simulink model "kinematics_model_Vw_working"  (R2020b)
settings: Solver=VariableStepAuto  StartTime=0.0  StopTime=100  RelTol=1e-3
values from neighbouring files (symbols this model uses):
  theta0 = 5*pi/180    (= 0.0872664625997)    [Kinematics_model.m]    (also in Path_Planning.m)
  x0 = 0    [Kinematics_model.m]    (also in Path_Planning.m)
  xd = x(length(x))    [APF.m]    (also in Kinematics_model.m = 20; Path_Planning.m = 6)
  y0 = 0    [Kinematics_model.m]    (also in Path_Planning.m)
  yd = y(length(y))    [APF.m]    (also in Kinematics_model.m = 15; Path_Planning.m = 7)
libraries: simulink_extras x1, mobileRoboticsLib x1
settings Model: Creator=Roooooomaaaaaaaaaaaa  LastModifiedBy=Roooooomaaaaaaaaaaaa

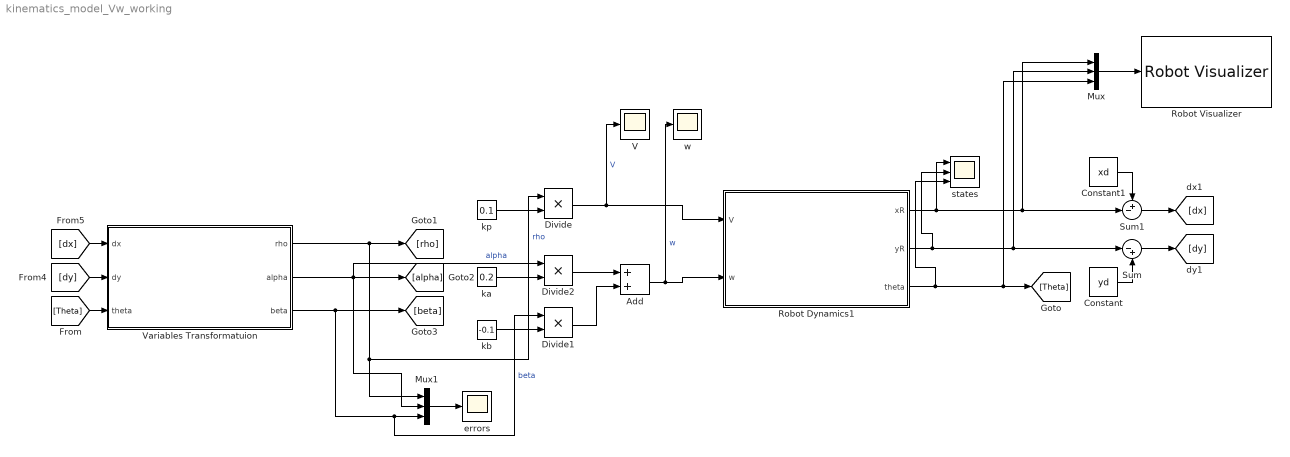
== system kinematics_model_Vw_working ==
  " Variables Transformatuion" : Subsystem
  Add : Sum
  Constant : Constant  Value=yd
  Constant1 : Constant  Value=xd
  Divide : Product  Inputs=**
  Divide1 : Product  Inputs=**
  Divide2 : Product  Inputs=**
  Mux : Mux  Inputs=3
  Mux1 : Mux  Inputs=3
  Robot Dynamics1 : Subsystem
  Robot Visualizer : mobileRoboticsLib/Environments/Robot Visualizer  robotRadius=r_w  showTrajectory=on  hasWaypoints=off  hasLidar=off  sensorOffset=[ 0, 0 ]  scanAngles=[ -pi/4, 0, pi/4 ]  hasObjDetector=off  objDetectorOffset=[ 0, 0 ]  objDetectorAngle=0  objDetectorFOV=pi/4  objDetectorMaxRange=5  objectColors=[ 1, 0, 0; 0, 1, 0; 0, 0, 1 ]  objectMarkers=s
  Sum : Sum  Inputs=|-+
  Sum1 : Sum  Inputs=+-|
  V : Scope
  errors : Scope
  ka : Constant  Value=0.2
  kb : Constant  Value=-0.1
  kp : Constant  Value=0.1
  states : Scope  NumInputPorts=3
  w : Scope
  wires:
  Mux/1 -> Robot Visualizer/1
  Divide1/1 -> Add/2
  Robot Dynamics1/2(yR) -> states/2, Sum/1, Mux/2
  Robot Dynamics1/3(theta) -> Mux/3, [Theta], states/3
  Divide2/1 -> Add/1
  [dy] -> " Variables Transformatuion"/2(dy)
  " Variables Transformatuion"/3(beta) -> [beta], Divide1/1, Mux1/3  "beta"
  " Variables Transformatuion"/2(alpha) -> Mux1/2, Divide2/1, [alpha]  "alpha"
  " Variables Transformatuion"/1(rho) -> Divide/1, Mux1/1, [rho]  "rho"
  kp/1 -> Divide/2
  ka/1 -> Divide2/2
  [Theta] -> " Variables Transformatuion"/3(theta)
  Sum1/1 -> [dx]
  Divide/1 -> V/1, Robot Dynamics1/1(V)  "V"
  Constant/1 -> Sum/2
  kb/1 -> Divide1/2
  Constant1/1 -> Sum1/1
  Sum/1 -> [dy]
  Robot Dynamics1/1(xR) -> states/1, Sum1/2, Mux/1
  Add/1 -> w/1, Robot Dynamics1/2(w)  "w"
  [dx] -> " Variables Transformatuion"/1(dx)
  Mux1/1 -> errors/1

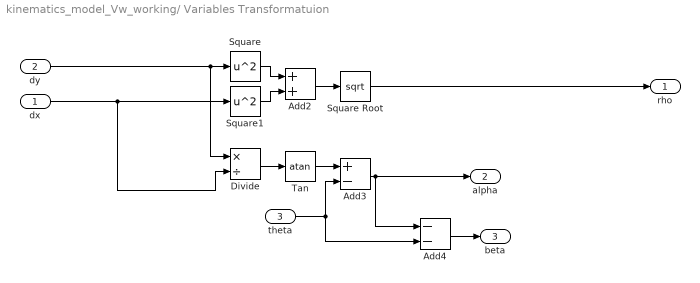
== system kinematics_model_Vw_working/ Variables Transformatuion ==
  dx : Inport
  dy : Inport  Port=2
  theta : Inport  Port=3
  Add2 : Sum
  Add3 : Sum  Inputs=+-
  Add4 : Sum  Inputs=--
  Divide : Product  Inputs=*/
  Square : Math  Operator=square  SaturateOnIntegerOverflow=on
  Square Root : Sqrt  SaturateOnIntegerOverflow=on
  Square1 : Math  Operator=square  SaturateOnIntegerOverflow=on
  Tan : Trigonometry  Operator=atan
  rho : Outport
  alpha : Outport  Port=2
  beta : Outport  Port=3
  wires:
  Square Root/1 -> rho/1
  Square1/1 -> Add2/2
  Square/1 -> Add2/1
  dx/1 -> Divide/2, Square1/1
  theta/1 -> Add3/2, Add4/2
  Divide/1 -> Tan/1
  Tan/1 -> Add3/1
  Add2/1 -> Square Root/1
  dy/1 -> Divide/1, Square/1
  Add3/1 -> alpha/1, Add4/1
  Add4/1 -> beta/1

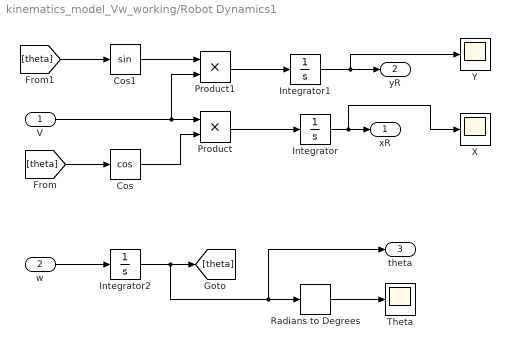
== system kinematics_model_Vw_working/Robot Dynamics1 ==
  V : Inport
  w : Inport  Port=2
  Cos : Trigonometry  Operator=cos
  Cos1 : Trigonometry
  Integrator : Integrator  InitialCondition=x0
  Integrator1 : Integrator  InitialCondition=y0
  Integrator2 : Integrator  InitialCondition=theta0
  Product : Product
  Product1 : Product
  Radians to Degrees : simulink_extras/Transformations/Radians to Degrees
  Theta : Scope
  X : Scope
  Y : Scope
  xR : Outport
  yR : Outport  Port=2
  theta : Outport  Port=3
  wires:
  Radians to Degrees/1 -> Theta/1
  Integrator1/1 -> Y/1, yR/1
  Cos/1 -> Product/2
  Integrator2/1 -> theta/1, Radians to Degrees/1, [theta]
  Product1/1 -> Integrator1/1
  Cos1/1 -> Product1/1
  Integrator/1 -> xR/1, X/1
  V/1 -> Product1/2, Product/1
  [theta] -> Cos/1
  [theta] -> Cos1/1
  Product/1 -> Integrator/1
  w/1 -> Integrator2/1
